simulink model "lab2"  (R2023b)
settings: Solver=VariableStepAuto  StartTime=0.0  StopTime=10.0  RelTol=1e-3
settings Model: Creator=Spedrik Webster  LastModifiedBy=Avijeet Jain

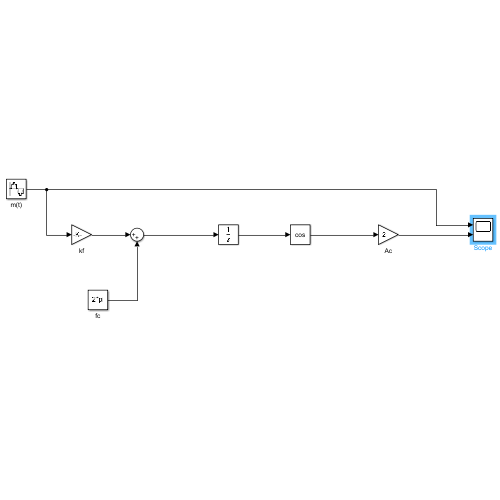
[thumbnail: Simulink's stored preview of the top-level diagram]
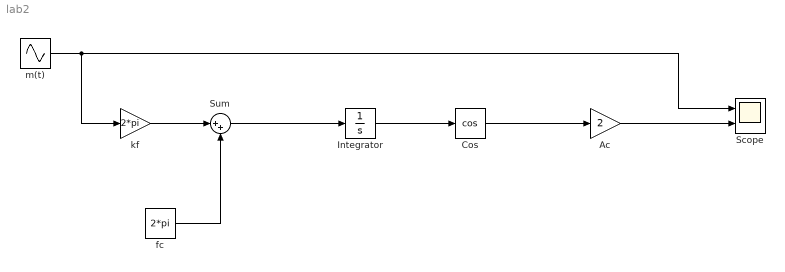
== system lab2 ==
  Ac : Gain  Gain=2
  Cos : Trigonometry  Operator=cos
  Integrator : Integrator
  Scope : Scope  NumInputPorts=2
  Sum : Sum  Inputs=|++
  fc : Constant  Value=2*pi
  kf : Gain  Gain=2*pi
  m(t) : Sin  Amplitude=2  Frequency=0.8  SampleTime=1/5000
  wires:
  m(t)/1 -> Scope/1, kf/1
  kf/1 -> Sum/1
  fc/1 -> Sum/2
  Ac/1 -> Scope/2
  Sum/1 -> Integrator/1
  Integrator/1 -> Cos/1
  Cos/1 -> Ac/1
